simulink model "ZkusLJu12w_Normalizovany_Zatizitelny"  (Simulink 7.8)
settings: Solver=ode45  StartTime=0.0  StopTime=inf  RelTol=1e-3
libraries: simulink x2
settings Model: Creator=frdu0449  LastModifiedBy=KRP

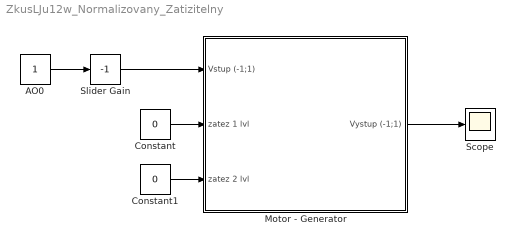
== system ZkusLJu12w_Normalizovany_Zatizitelny ==
  AO0 : Constant
  Constant : Constant  Value=0
  Constant1 : Constant  Value=0
  Motor - Generator : Subsystem
  Scope : Scope
      settings: YMin=-0.43  YMax=-0.24
  Slider Gain : simulink/Math Operations/Slider Gain  low=-1  gain=-1  high=1
  wires:
  AO0/1 -> Slider Gain/1
  Constant/1 -> Motor - Generator/2(zatez 1 lvl)
  Constant1/1 -> Motor - Generator/3(zatez 2 lvl)
  Slider Gain/1 -> Motor - Generator/1(Vstup (-1;1))
  Motor - Generator/1(Vystup (-1;1)) -> Scope/1

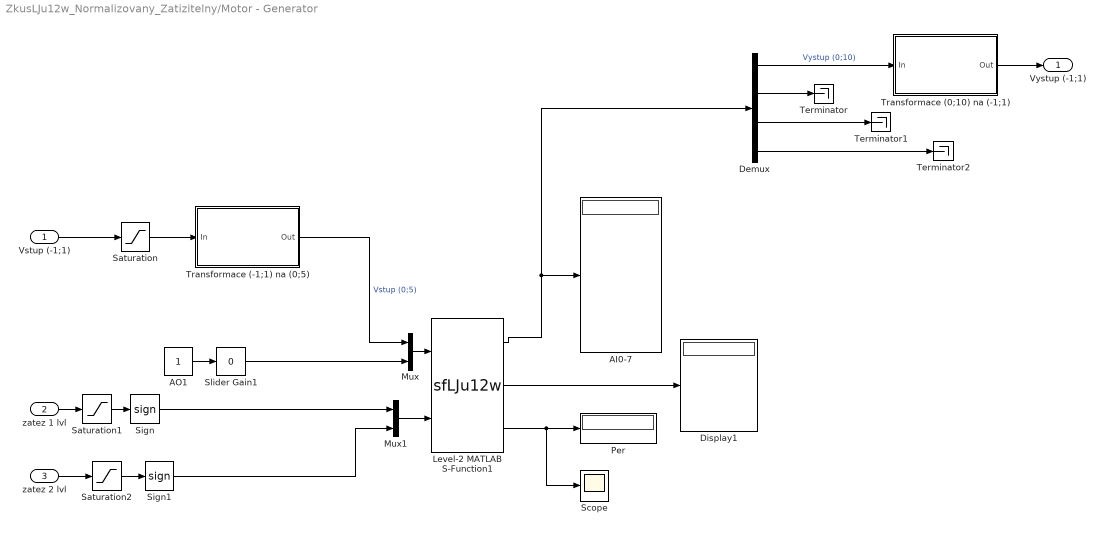
== system ZkusLJu12w_Normalizovany_Zatizitelny/Motor - Generator ==
  Vstup (-1;1) : Inport
  zatez 1 lvl : Inport  Port=2
  zatez 2 lvl : Inport  Port=3
  AI0-7 : Display
  AO1 : Constant
  Demux : Demux
  Display1 : Display
  Level-2 MATLAB S-Function1 : M-S-Function  FunctionName=sfLJu12w  Parameters=0,0.1,[0,0,1,1],[0,1,2,3],[0,0,0,0]
  Mux : Mux  Inputs=2
  Mux1 : Mux  Inputs=2
  Per : Display
  Saturation : Saturate  UpperLimit=1  LowerLimit=-1
  Saturation1 : Saturate  UpperLimit=1  LowerLimit=0
  Saturation2 : Saturate  UpperLimit=1  LowerLimit=0
  Scope : Scope
      settings: YMin=0.075  YMax=0.3
  Sign : Signum
  Sign1 : Signum
  Slider Gain1 : simulink/Math Operations/Slider Gain  low=0  gain=0  high=5
  Terminator : Terminator
  Terminator1 : Terminator
  Terminator2 : Terminator
  Transformace (-1;1) na (0;5) : Subsystem
  Transformace (0;10) na (-1;1) : Subsystem
  Vystup (-1;1) : Outport
  wires:
  AO1/1 -> Slider Gain1/1
  Level-2 MATLAB S-Function1/1 -> AI0-7/1, Demux/1
  Vstup (-1;1)/1 -> Saturation/1
  Slider Gain1/1 -> Mux/2
  Transformace (-1;1) na (0;5)/1(Out) -> Mux/1  "Vstup (0;5)"
  Demux/2 -> Terminator/1
  Demux/3 -> Terminator1/1
  Demux/4 -> Terminator2/1
  Demux/1 -> Transformace (0;10) na (-1;1)/1(In)  "Vystup (0;10)"
  Transformace (0;10) na (-1;1)/1(Out) -> Vystup (-1;1)/1
  Saturation/1 -> Transformace (-1;1) na (0;5)/1(In)
  Mux/1 -> Level-2 MATLAB S-Function1/1
  Level-2 MATLAB S-Function1/3 -> Per/1, Scope/1
  Level-2 MATLAB S-Function1/2 -> Display1/1
  Mux1/1 -> Level-2 MATLAB S-Function1/2
  zatez 1 lvl/1 -> Saturation1/1
  zatez 2 lvl/1 -> Saturation2/1
  Saturation1/1 -> Sign/1
  Sign/1 -> Mux1/1
  Sign1/1 -> Mux1/2
  Saturation2/1 -> Sign1/1

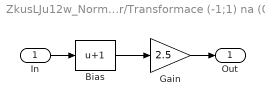
== system ZkusLJu12w_Normalizovany_Zatizitelny/Motor - Generator/Transformace (-1;1) na (0;5) ==
  In : Inport
  Bias : Bias  Bias=1
  Gain : Gain  Gain=2.5
  Out : Outport
  wires:
  Bias/1 -> Gain/1
  In/1 -> Bias/1
  Gain/1 -> Out/1

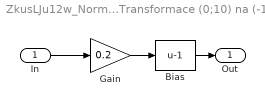
== system ZkusLJu12w_Normalizovany_Zatizitelny/Motor - Generator/Transformace (0;10) na (-1;1) ==
  In : Inport
  Bias : Bias  Bias=-1
  Gain : Gain  Gain=0.2
  Out : Outport
  wires:
  Gain/1 -> Bias/1
  In/1 -> Gain/1
  Bias/1 -> Out/1
